simulink subsystem "HighLevelController"  (R2022b)
settings: Solver=VariableStepAuto  StartTime=0.0  StopTime=10.0  RelTol=1e-3
undefined symbols (not defined in the file): ProjectExample
settings Model: Creator=Ilya_Andriyanov  LastModifiedBy=user

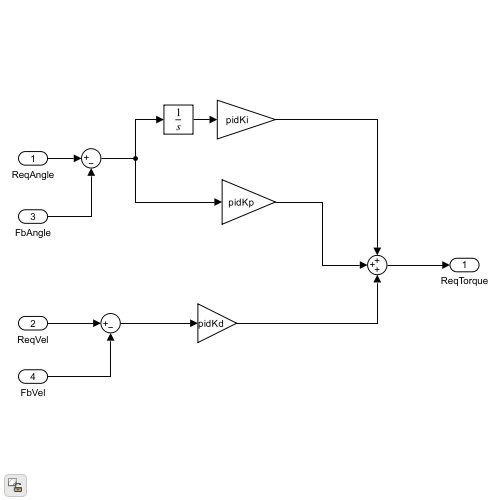
[thumbnail: Simulink's stored preview of the top-level diagram]
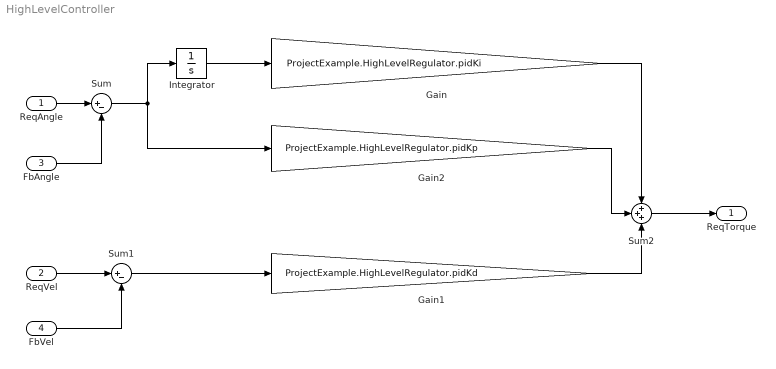
== system HighLevelController ==
  ReqAngle : Inport
  ReqVel : Inport  Port=2
  FbAngle : Inport  Port=3
  FbVel : Inport  Port=4
  Gain : Gain  Gain=ProjectExample.HighLevelRegulator.pidKi
  Gain1 : Gain  Gain=ProjectExample.HighLevelRegulator.pidKd
  Gain2 : Gain  Gain=ProjectExample.HighLevelRegulator.pidKp
  Integrator : Integrator
  Sum : Sum  Inputs=|+-
  Sum1 : Sum  Inputs=|+-
  Sum2 : Sum  Inputs=+++
  ReqTorque : Outport
  wires:
  ReqAngle/1 -> Sum/1
  FbAngle/1 -> Sum/2
  ReqVel/1 -> Sum1/1
  FbVel/1 -> Sum1/2
  Sum/1 -> Integrator/1, Gain2/1
  Sum2/1 -> ReqTorque/1
  Integrator/1 -> Gain/1
  Gain/1 -> Sum2/1
  Gain2/1 -> Sum2/2
  Sum1/1 -> Gain1/1
  Gain1/1 -> Sum2/3
